simulink model "pipeline_sar_adc"  (R2026a)
settings: Solver=FixedStepDiscrete  FixedStep=1e-10
values from neighbouring files (symbols this model uses):
  bit_1st = 6    [script_MonteCarlo.m]    (also in script_MonteCarlo_v2.m; script_spectrum.m; script_spectrum_v2.m)
  bit_2nd = 9    [script_MonteCarlo.m]    (also in script_MonteCarlo_v2.m; script_spectrum.m; script_spectrum_v2.m)
  CMPno_1st = 0    [script_MonteCarlo.m]    (also in script_MonteCarlo_v2.m = 0.0001; script_spectrum.m; script_spectrum_v2.m)
  CMPno_2nd = 0    [script_MonteCarlo.m]    (also in script_MonteCarlo_v2.m = 0.001; script_spectrum.m; script_spectrum_v2.m)
  CMPoff_1st = 0    [script_MonteCarlo.m]    (also in script_MonteCarlo_v2.m = 0.001; script_spectrum.m; script_spectrum_v2.m)
  CMPoff_2nd = 0    [script_MonteCarlo.m]    (also in script_MonteCarlo_v2.m = 0.001; script_spectrum.m; script_spectrum_v2.m)
  DAC_1st = DAC_1st_scaled(1 : (bit_1st + 1)) / (2^bit_1st)    [script_MonteCarlo.m]    (also in script_MonteCarlo_v2.m; script_spectrum.m; script_spectrum_v2.m)
  DAC_2nd = 0    [script_MonteCarlo.m]    (also in script_MonteCarlo_v2.m; script_spectrum.m; script_spectrum_v2.m)
  fin = (M / N) * fs    (= 488281.25)    [script_MonteCarlo.m]    (also in script_MonteCarlo_v2.m; script_spectrum.m; script_spectrum_v2.m)
  fs = 100e6    (= 100000000)    [script_MonteCarlo.m]    (also in script_MonteCarlo_v2.m; script_spectrum.m; script_spectrum_v2.m)
  Vin = 0.95    [script_MonteCarlo.m]    (also in script_MonteCarlo_v2.m; script_parametric_analysis.m = Vin_array(idx); script_spectrum.m; script_spectrum_v2.m)
settings Model: Creator=오지훈  LastModifiedBy=오지훈

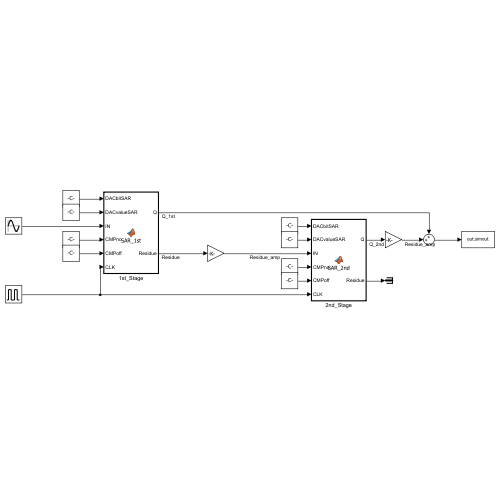
[thumbnail: Simulink's stored preview of the top-level diagram]
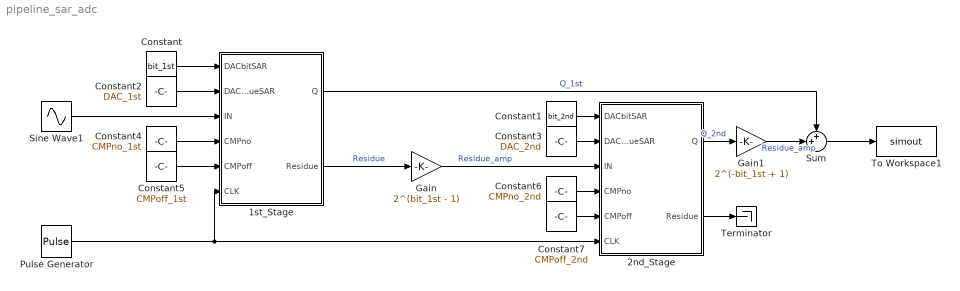
== system pipeline_sar_adc ==
  1st_Stage : MATLAB Function  TreatAsAtomicUnit=on
  2nd_Stage : MATLAB Function  TreatAsAtomicUnit=on
  Constant : Constant  Value=bit_1st
  Constant1 : Constant  Value=bit_2nd
  Constant2 : Constant  Value=DAC_1st
  Constant3 : Constant  Value=DAC_2nd
  Constant4 : Constant  Value=CMPno_1st
  Constant5 : Constant  Value=CMPoff_1st
  Constant6 : Constant  Value=CMPno_2nd
  Constant7 : Constant  Value=CMPoff_2nd
  Gain : Gain  Gain=2^(bit_1st - 1)
  Gain1 : Gain  Gain=2^(-bit_1st + 1)
  Pulse Generator : DiscretePulseGenerator  PulseType=Time based  Period=1/fs  PulseWidth=50
  Sine Wave1 : Sin  Amplitude=Vin  Frequency=2*pi*fin  SampleTime=0
  Sum : Sum  Inputs=++|
  Terminator : Terminator
  To Workspace1 : ToWorkspace  VariableName=simout  SaveFormat=Timeseries  SampleTime=1/fs
  wires:
  Constant6/1 -> 2nd_Stage/4(CMPno)
  Constant5/1 -> 1st_Stage/5(CMPoff)
  Constant3/1 -> 2nd_Stage/2(DACvalueSAR)
  Constant4/1 -> 1st_Stage/4(CMPno)
  1st_Stage/2(Residue) -> Gain/1  "Residue"
  Sine Wave1/1 -> 1st_Stage/3(IN)
  Pulse Generator/1 -> 2nd_Stage/6(CLK), 1st_Stage/6(CLK)
  Constant2/1 -> 1st_Stage/2(DACvalueSAR)
  Gain/1 -> 2nd_Stage/3(IN)  "Residue_amp"
  Constant7/1 -> 2nd_Stage/5(CMPoff)
  Constant1/1 -> 2nd_Stage/1(DACbitSAR)
  2nd_Stage/2(Residue) -> Terminator/1
  Constant/1 -> 1st_Stage/1(DACbitSAR)
  Sum/1 -> To Workspace1/1
  Gain1/1 -> Sum/2  "Residue_amp"
  2nd_Stage/1(Q) -> Gain1/1  "Q_2nd"
  1st_Stage/1(Q) -> Sum/1  "Q_1st"

== matlab function pipeline_sar_adc/1st_Stage ==
  data: DACbitSAR input; Q output; DACvalueSAR input; IN input; CMPno input; CMPoff input; Residue output; CLK input
function [Q, Residue] = SAR_1st(DACbitSAR, DACvalueSAR, IN, CMPno, CMPoff, CLK)
persistent last_CLK Q_hold Residue_hold

if isempty(last_CLK)
    last_CLK = 0;
    Q_hold = 0;
    Residue_hold = 0;
end

if (last_CLK == 0) && (CLK == 1)
    
    current_residue = IN; 
    Q_partial_sum = 0;    % ★ Partial sum을 누적할 변수 초기화
    len_DAC = length(DACvalueSAR); 
    
    for i = 1:DACbitSAR
        CMP_threshold = CMPno * randn(1) + CMPoff;
        
        current_idx = len_DAC - i + 1; 
        current_dac = DACvalueSAR(current_idx);
        
        % 각 비트 자리에 해당하는 이진 가중치 (1, 0.5, 0.25, 0.125 ...)
        bit_weight = 2^(-(i-1)); 
        
        if current_residue >= CMP_threshold
            current_residue = current_residue - current_dac;
            % ★ 비트가 1일 때, 가중치(bit_weight)를 partial sum에 바로 누적
            Q_partial_sum = Q_partial_sum + 1 * bit_weight;
        else
            current_residue = current_residue + current_dac;
            % 비트가 0일 때는 0 * bit_weight 이므로 누적 생략 (혹은 +0)
        end
    end
    
    % ★ 최종 스케일링: [2 곱하기]를 빼고 [1만 빼는] 규칙 적용
    % Virtuoso 수식의 ((VT(MSB) + VT(MSB-1)/2 + ...) - 1) 과 완벽히 매칭됩니다.
    Q_hold = Q_partial_sum - 1;
    
    Residue_hold = current_residue;
end

Q = Q_hold;
Residue = Residue_hold;
last_CLK = CLK;
end

== matlab function pipeline_sar_adc/2nd_Stage ==
  data: DACbitSAR input; Q output; DACvalueSAR input; IN input; CMPno input; CMPoff input; Residue output; CLK input
function [Q, Residue] = SAR_2nd(DACbitSAR, DACvalueSAR, IN, CMPno, CMPoff, CLK)
persistent last_CLK Q_hold Residue_hold

if isempty(last_CLK)
    last_CLK = 0;
    Q_hold = 0;
    Residue_hold = 0;
end

if (last_CLK == 0) && (CLK == 1)
    
    current_residue = IN; 
    Q_partial_sum = 0;    % ★ Partial sum을 누적할 변수 초기화
    len_DAC = length(DACvalueSAR); 
    
    for i = 1:DACbitSAR
        CMP_threshold = CMPno * randn(1) + CMPoff;
        
        current_idx = len_DAC - i + 1; 
        current_dac = DACvalueSAR(current_idx);
        
        % 각 비트 자리에 해당하는 이진 가중치 (1, 0.5, 0.25, 0.125 ...)
        bit_weight = 2^(-(i-1)); 
        
        if current_residue >= CMP_threshold
            current_residue = current_residue - current_dac;
            % ★ 비트가 1일 때, 가중치(bit_weight)를 partial sum에 바로 누적
            Q_partial_sum = Q_partial_sum + 1 * bit_weight;
        else
            current_residue = current_residue + current_dac;
            % 비트가 0일 때는 0 * bit_weight 이므로 누적 생략 (혹은 +0)
        end
    end
    
    % ★ 최종 스케일링: [2 곱하기]를 빼고 [1만 빼는] 규칙 적용
    % Virtuoso 수식의 ((VT(MSB) + VT(MSB-1)/2 + ...) - 1) 과 완벽히 매칭됩니다.
    Q_hold = Q_partial_sum - 1;
    
    Residue_hold = current_residue;
end

Q = Q_hold;
Residue = Residue_hold;
last_CLK = CLK;
end
